simulink model "linearizedTurbine_mdl"  (R2022b)
settings: Solver=ode4  StartTime=0.0  StopTime=0.1  FixedStep=.001  RelTol=1e-3
undefined symbols (not defined in the file): F, G_theta, sys
settings Model: Creator=mo780715  LastModifiedBy=mo780715

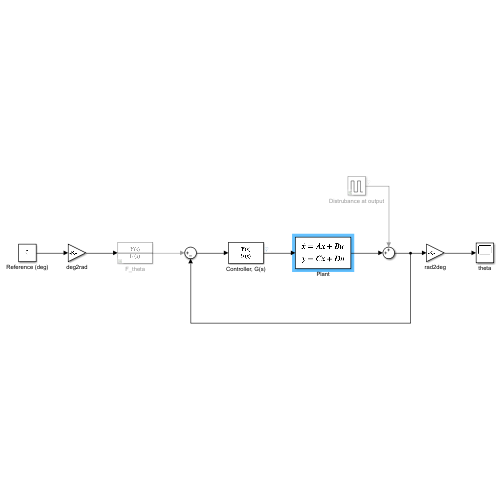
[thumbnail: Simulink's stored preview of the top-level diagram]
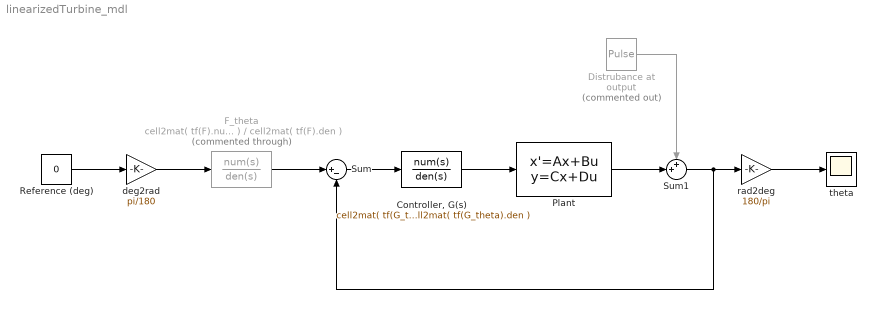
== system linearizedTurbine_mdl ==
  "Controller, G(s)" : TransferFcn  Numerator=cell2mat( tf(G_theta).num )  Denominator=cell2mat( tf(G_theta).den )  ContinuousStateAttributes='theta'
  Distrubance at output : DiscretePulseGenerator  Commented=on  PulseType=Time based  Amplitude=0*pi/180  Period=1e6  PulseWidth=1/1e6  PhaseDelay=0.5
  F_theta : TransferFcn  Commented=through  Numerator=cell2mat( tf(F).num )  Denominator=cell2mat( tf(F).den )
  Plant : StateSpace  A=sys.A  B=sys.B  C=sys.C  D=sys.D  InitialCondition=[0 5/180*pi /-0.5]  ContinuousStateAttributes='theta'
  Reference (deg) : Constant  Value=0
  Sum : Sum  Inputs=|+-
  Sum1 : Sum  Inputs=++|
  deg2rad : Gain  Gain=pi/180
  rad2deg : Gain  Gain=180/pi
  theta : Scope
  wires:
  rad2deg/1 -> theta/1
  Reference (deg)/1 -> deg2rad/1
  F_theta/1 -> Sum/1
  Sum/1 -> "Controller, G(s)"/1
  deg2rad/1 -> F_theta/1
  Plant/1 -> Sum1/2
  Sum1/1 -> Sum/2, rad2deg/1
  Distrubance at output/1 -> Sum1/1
  "Controller, G(s)"/1 -> Plant/1
